simulink model "TMATS_Example_1"  (R2019a)
settings: Solver=FixedStepDiscrete  StartTime=0.0  StopTime=10.0  RelTol=1e-3
libraries: Lib_Solve_SSNRSolverJC_TMATS x1
settings Model: Creator=bbraunj  LastModifiedBy=bbraunj

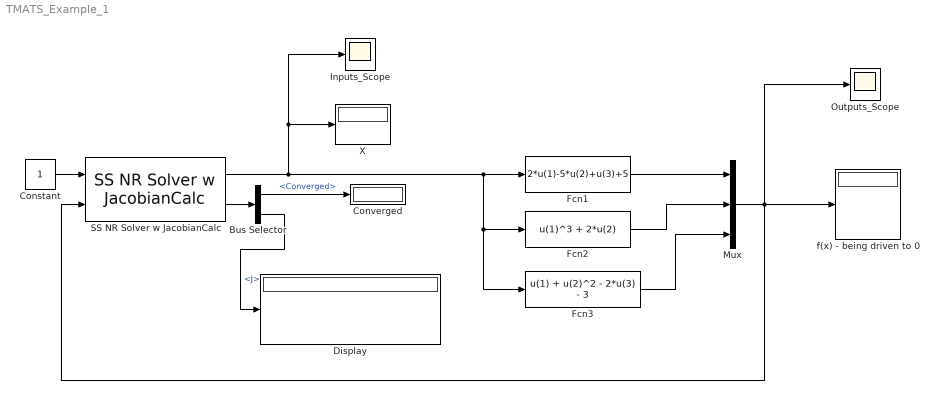
== system TMATS_Example_1 ==
  Bus Selector : BusSelector  OutputSignals=Converged,J
  Constant : Constant
  Converged : Display
  Display : Display
  Fcn1 : Fcn  Expr=2*u(1)-5*u(2)+u(3)+5
  Fcn2 : Fcn  Expr=u(1)^3 + 2*u(2)
  Fcn3 : Fcn  Expr=u(1) + u(2)^2 - 2*u(3) - 3
  Inputs_Scope : Scope
  Mux : Mux  Inputs=3
  Outputs_Scope : Scope
  SS NR Solver w JacobianCalc : Lib_Solve_SSNRSolverJC_TMATS/SS NR Solver w JacobianCalc  SJac_Per_M=3  SNR_IC_M=3  SNR_DX_M=5  SNR_Mx_M=100000  SNR_Mn_M=0.00001  SJacobianAttempts_M=20  Cond_Limits_M=0.0001
  X : Display
  f(x) - being driven to 0 : Display
  wires:
  SS NR Solver w JacobianCalc/1 -> Inputs_Scope/1, X/1, Fcn3/1, Fcn2/1, Fcn1/1
  SS NR Solver w JacobianCalc/2 -> Bus Selector/1
  Fcn2/1 -> Mux/2
  Fcn3/1 -> Mux/3
  Mux/1 -> Outputs_Scope/1, SS NR Solver w JacobianCalc/2, f(x) - being driven to 0/1
  Bus Selector/1 -> Converged/1  "<Converged>"
  Bus Selector/2 -> Display/1  "<J>"
  Fcn1/1 -> Mux/1
  Constant/1 -> SS NR Solver w JacobianCalc/1
